simulink model "ego_1"  (R2024b)
settings: Solver=FixedStepAuto  StartTime=0.0  StopTime=5  RelTol=1e-3
settings Model: Creator=DELL  LastModifiedBy=DELL

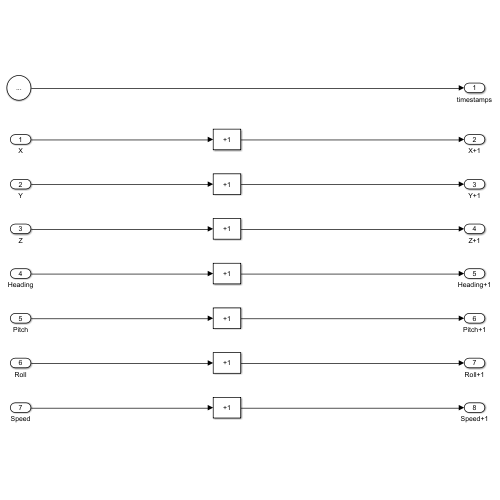
[thumbnail: Simulink's stored preview of the top-level diagram]
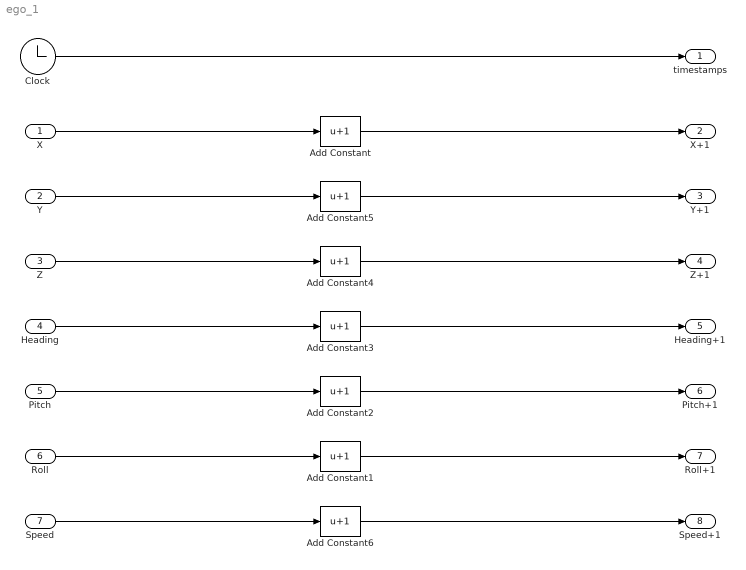
== system ego_1 ==
  X : Inport  Tag=X
  Y : Inport  Tag=Y  Port=2
  Z : Inport  Tag=Z  Port=3
  Heading : Inport  Tag=Heading  Port=4
  Pitch : Inport  Tag=Pitch  Port=5
  Roll : Inport  Tag=Roll  Port=6
  Speed : Inport  Tag=Speed  Port=7
  Add Constant{,1..6} (7 alike) : Bias  Bias=1  SaturateOnIntegerOverflow=off
  Clock : Clock
  timestamps : Outport
  X+1 : Outport  Port=2
  Y+1 : Outport  Port=3
  Z+1 : Outport  Port=4
  Heading+1 : Outport  Port=5
  Pitch+1 : Outport  Port=6
  Roll+1 : Outport  Port=7
  Speed+1 : Outport  Port=8
  wires:
  Clock/1 -> timestamps/1
  X/1 -> Add Constant/1
  Add Constant/1 -> X+1/1
  Y/1 -> Add Constant5/1
  Z/1 -> Add Constant4/1
  Add Constant4/1 -> Z+1/1
  Add Constant5/1 -> Y+1/1
  Heading/1 -> Add Constant3/1
  Add Constant3/1 -> Heading+1/1
  Pitch/1 -> Add Constant2/1
  Add Constant2/1 -> Pitch+1/1
  Roll/1 -> Add Constant1/1
  Add Constant1/1 -> Roll+1/1
  Speed/1 -> Add Constant6/1
  Add Constant6/1 -> Speed+1/1
